simulink model "PWM"  (R2014a)
settings: Solver=ode8  StartTime=0.0  StopTime=5  FixedStep=5e-6  RelTol=1e-3
values from neighbouring files (symbols this model uses):
  C = 1/((2*pi*fc)^2*L*10^-3)    [PWWW.m]
  L = input('Valor do Indutor (mH): ')    [PWM.m]    (also in PWWW.m = input('Digite o valor de L(mH): '))
libraries: powerlib x13, powerlib_meascontrol x1
settings Model: Creator=Luciano  LastModifiedBy=Luciano

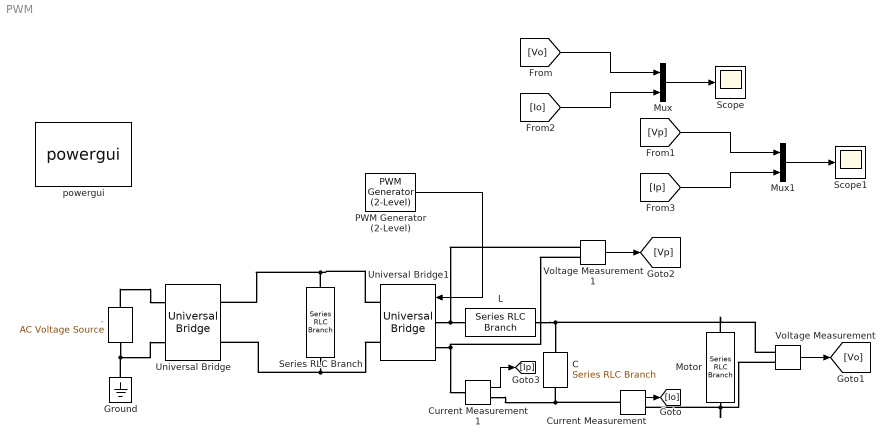
== system PWM ==
  ". " : powerlib/Electrical Sources/AC Voltage Source  Amplitude=100  Phase=0  Frequency=60  SampleTime=0  Measurements=None
  C : powerlib/Elements/Series RLC Branch  LConnTagsString=__new0  RConnTagsString=__new0  BranchType=C  Resistance=0  Inductance=0  SetiL0=off  InitialCurrent=0  Capacitance=C  Setx0=off  InitialVoltage=0  Measurements=None
  Current Measurement : powerlib/Measurements/Current Measurement  PhasorSimulation=off  OutputType=Complex  PSBequivalent=0
  Current Measurement1 : powerlib/Measurements/Current Measurement  PhasorSimulation=off  OutputType=Complex  PSBequivalent=0
  Ground : powerlib/Elements/Ground  LConnTagsString=a
  L : powerlib/Elements/Series RLC Branch  LConnTagsString=__new0  RConnTagsString=__new0  BranchType=L  Resistance=0  Inductance=L  SetiL0=off  InitialCurrent=0  Capacitance=1e-6  Setx0=off  InitialVoltage=0  Measurements=None
  Motor : powerlib/Elements/Series RLC Branch  LConnTagsString=__new0  RConnTagsString=__new0  BranchType=RL  Resistance=10  Inductance=100e-3  SetiL0=off  InitialCurrent=0  Capacitance=1e-6  Setx0=off  InitialVoltage=0  Measurements=None
  Mux : Mux  Inputs=2
  Mux1 : Mux  Inputs=2
  PWM Generator (2-Level) : powerlib_meascontrol/Pulse & Signal Generators/PWM Generator (2-Level)  ModulatorType=Single-phase full-bridge (4 pulses)  ModulatorMode=Unsynchronized  nF=27  Fc=27*60  ModulatingSignals=on  m=0.8  Freq=60  Phase=0  Ts=5e-6
  Scope : Scope
      settings: TimeRange=5
  Scope1 : Scope
      settings: TimeRange=5  YMin=-500  YMax=500
  Series RLC Branch : powerlib/Elements/Series RLC Branch  LConnTagsString=__new0  RConnTagsString=__new0  BranchType=C  Resistance=0  Inductance=0  SetiL0=off  InitialCurrent=0  Capacitance=1e-6  Setx0=off  InitialVoltage=0  Measurements=None
  Universal Bridge : powerlib/Power Electronics/Universal Bridge  Arms=2  SnubberResistance=1e5  SnubberCapacitance=inf  Device=Diodes  Ron=1e-3  Lon=0  ForwardVoltages="[  0  0  ]"  ForwardVoltage=0  GTOparameters=[ 10e-6 , 20e-6 ]  IGBTparameters=[ 1e-6 , 2e-6 ]  Measurements=None  Measurements_2=None  converterType=Rectifier
  Universal Bridge1 : powerlib/Power Electronics/Universal Bridge  Arms=2  SnubberResistance=1e5  SnubberCapacitance=inf  Device=IGBT / Diodes  Ron=1e-3  Lon=0  ForwardVoltages="[  0  0  ]"  ForwardVoltage=0  GTOparameters=[ 10e-6 , 20e-6 ]  IGBTparameters=[ 1e-6 , 2e-6 ]  Measurements=None  Measurements_2=None  converterType=Rectifier
  Voltage Measurement : powerlib/Measurements/Voltage Measurement  PhasorSimulation=off  OutputType=Complex  PSBequivalent=0
  Voltage Measurement1 : powerlib/Measurements/Voltage Measurement  PhasorSimulation=off  OutputType=Complex  PSBequivalent=0
  powergui : powerlib/powergui  Priority=1  SimulationMode=Discrete  SolverType=Tustin  SampleTime=5e-6  frequency=60  SPID=off  DisableSnubberDevices=off  DisableRonSwitches=off  DisableVfSwitches=off  SwTol=0  Interpol=off  DisplayEquations=off  Ts=0  methode=off  frequencyindice=60  Pbase=100e6  ErrMax=1e-4  Iterations=50  UnitsV=kV  UnitsW=MW  FunctionMessages=off  echomessages=off  HookPort=off  EnableUseOfTLC=off  x0status=blocks  RestoreLinks=warning  ResistiveCurrentMeasurement=off  Frange=[0:2:500]  Ylog=off  Xlog=on  ShowGrid=off  save=off  variable=ZData  structure=0  ZoomFFT=off  StartTime=0.0  cycles=1  DisplayStyle=1  fundamental=60  FreqAxis=off  MaxFrequency=1000  frequencyindicesteady=1  RmsSteady=1  display=off
  wires:
  PWM Generator (2-Level)/1 -> Universal Bridge1/1
  Current Measurement/1 -> [Io]
  Voltage Measurement/1 -> [Vo]
  [Vo] -> Mux/1
  Mux/1 -> Scope/1
  [Io] -> Mux/2
  Voltage Measurement1/1 -> [Vp]
  Current Measurement1/1 -> [Ip]
  [Vp] -> Mux1/1
  Mux1/1 -> Scope1/1
  [Ip] -> Mux1/2
  connections:
  ". "/RConn1 -- Universal Bridge/LConn1
  ". "/LConn1 -- Ground/LConn1 -- Universal Bridge/LConn2
  Universal Bridge1/RConn1 -- Series RLC Branch/LConn1 -- Universal Bridge/RConn1
  Universal Bridge1/RConn2 -- Series RLC Branch/RConn1 -- Universal Bridge/RConn2
  Universal Bridge1/LConn1 -- Voltage Measurement1/LConn1 -- L/LConn1
  L/RConn1 -- Voltage Measurement/LConn1 -- Motor/RConn1 -- C/LConn1
  Motor/LConn1 -- Current Measurement/RConn1 -- Voltage Measurement/LConn2
  Current Measurement/LConn1 -- Current Measurement1/RConn1 -- C/RConn1
  Universal Bridge1/LConn2 -- Current Measurement1/LConn1 -- Voltage Measurement1/LConn2
